simulink model "w2p4_model"  (R2020a)
settings: Solver=VariableStepAuto  StartTime=0.0  StopTime=0.2  RelTol=1e-3
model workspace (MAT data in the model file):
  J = Simulink.Parameter
  J.Value = 3.2284e-06
  J.DataType = 'auto'
  J.Dimensions = [1 1]
  L = Simulink.Parameter
  L.Value = 2.75e-06
  L.DataType = 'auto'
  L.Dimensions = [1 1]
  R = Simulink.Parameter
  R.Value = 4
  R.DataType = 'auto'
  R.Dimensions = [1 1]
  b = Simulink.Parameter
  b.Value = 3.5077e-06
  b.DataType = 'auto'
  b.Dimensions = [1 1]
  kd = Simulink.Parameter
  kd.Value = 200
  kd.DataType = 'auto'
  kd.Dimensions = [1 1]
  ke = Simulink.Parameter
  ke.Value = 0.0274
  ke.DataType = 'auto'
  ke.Dimensions = [1 1]
  ki = Simulink.Parameter
  ki.Value = 350
  ki.DataType = 'auto'
  ki.Dimensions = [1 1]
  kp = Simulink.Parameter
  kp.Value = 800
  kp.DataType = 'auto'
  kp.Dimensions = [1 1]
  kt = Simulink.Parameter
  kt.Value = 0.0274
  kt.DataType = 'auto'
  kt.Dimensions = [1 1]
settings Model: Creator=avn19  LastModifiedBy=avn19

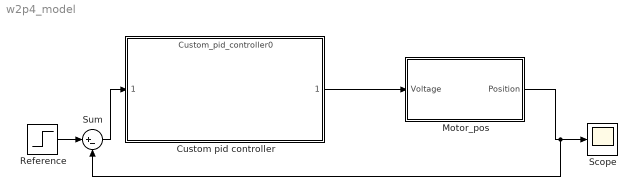
== system w2p4_model ==
  Custom pid controller : ModelReference  ModelNameDialog=Custom_pid_controller0  SimulationMode=Normal  ModelReferenceVersion=1.1
  Motor_pos : Subsystem
  Reference : Step  Time=0  SampleTime=0
  Scope : Scope
  Sum : Sum  Inputs=|+-
  wires:
  Motor_pos/1(Position) -> Sum/2, Scope/1
  Custom pid controller/1 -> Motor_pos/1(Voltage)
  Reference/1 -> Sum/1
  Sum/1 -> Custom pid controller/1

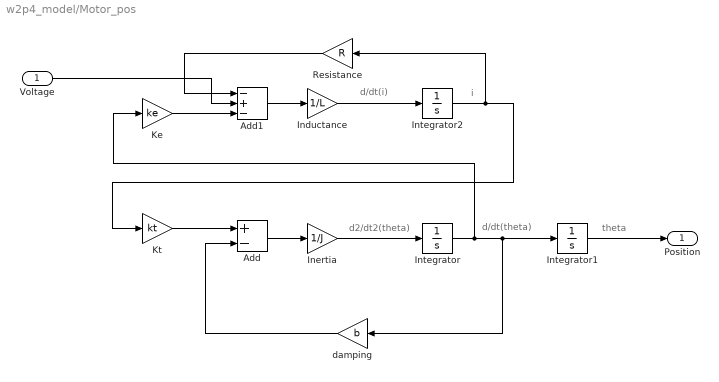
== system w2p4_model/Motor_pos ==
  note: theta
  note: d/dt(theta)
  note: d2/dt2(theta)
  note: d/dt(i)
  note: i
  Voltage : Inport
  Add : Sum  Inputs=+-
  Add1 : Sum  Inputs=-+-
  Inductance : Gain  Gain=1/L
  Inertia : Gain  Gain=1/J
  Integrator : Integrator
  Integrator1 : Integrator
  Integrator2 : Integrator
  Ke : Gain  Gain=ke
  Kt : Gain  Gain=kt
  Resistance : Gain  Gain=R
  damping : Gain  Gain=b
  Position : Outport
  wires:
  Add1/1 -> Inductance/1
  Ke/1 -> Add1/3
  Resistance/1 -> Add1/1
  Kt/1 -> Add/1
  damping/1 -> Add/2
  Add/1 -> Inertia/1
  Voltage/1 -> Add1/2
  Integrator1/1 -> Position/1
  Integrator/1 -> Integrator1/1, damping/1, Ke/1
  Integrator2/1 -> Kt/1, Resistance/1
  Inductance/1 -> Integrator2/1
  Inertia/1 -> Integrator/1
